simulink model "sampleModel1941_4_sub_sub_sub"  (R2023a)
settings: Solver=VariableStepAuto  StartTime=0.0  StopTime=10.0  RelTol=1e-3
libraries: hdlsllib x3, simulink x1
settings Model: Creator=user1  LastModifiedBy=user1
settings OptimizationCC: BlockReduction=off  ConditionallyExecuteInputs=off

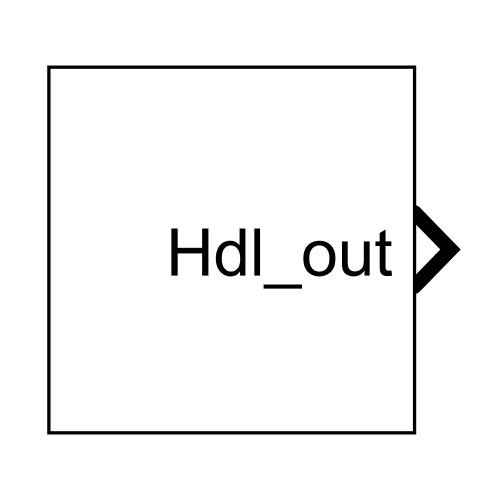
[thumbnail: Simulink's stored preview of the top-level diagram]
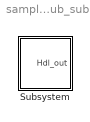
== system sampleModel1941_4_sub_sub_sub ==
  Subsystem : Subsystem

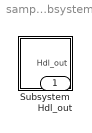
== system sampleModel1941_4_sub_sub_sub/Subsystem ==
  Subsystem : Subsystem
  Hdl_out : Outport  OutDataTypeStr=uint8

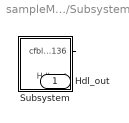
== system sampleModel1941_4_sub_sub_sub/Subsystem/Subsystem ==
  Subsystem : Subsystem
  Hdl_out : Outport  OutDataTypeStr=uint8
  wires:
  Subsystem/1(cfblk136) -> Hdl_out/1

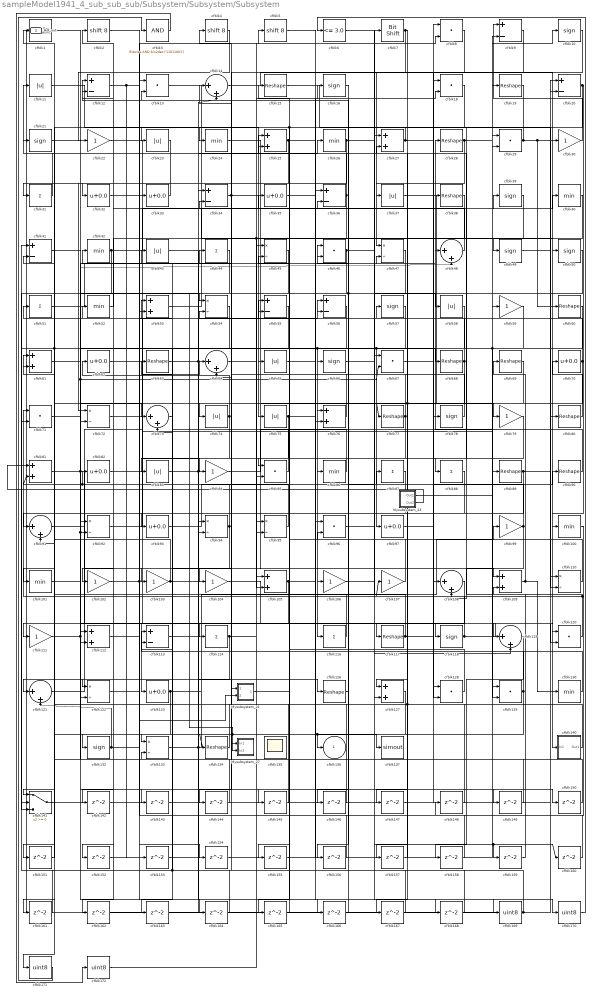
== system sampleModel1941_4_sub_sub_sub/Subsystem/Subsystem/Subsystem ==
  Mysubsystem_21 : Subsystem  TreatAsAtomicUnit=on  RTWFcnName=Mysubsystem_21
      settings: RTWFcnNameOpts=User specified  RTWFileNameOpts=Use function name
  Mysubsystem_23 : Subsystem  TreatAsAtomicUnit=on  RTWFcnName=Mysubsystem_23
      settings: RTWFcnNameOpts=User specified  RTWFileNameOpts=Use function name
  Mysubsystem_27 : Subsystem  TreatAsAtomicUnit=on  RTWFcnName=Mysubsystem_27
      settings: RTWFcnNameOpts=User specified  RTWFileNameOpts=Use function name
  cfblk1 : hdlsllib/Logic and Bit Operations/Detect Rise Nonnegative  vinit=0  OutDataTypeStr=uint8
  cfblk{10,16,21,39,49..50,57,66,78,118,132} (11 alike) : Signum
  cfblk{24,26,40,42,52,86,100..101,130} (9 alike) : MinMax  OutDataTypeStr=uint8
  cfblk{22,30,59,79,84,99,102..104,106..107,111} (12 alike) : Gain  OutDataTypeStr=uint8
  cfblk{25,27,53,61,76,81,105,109,112,127} (10 alike) : Sum  OutDataTypeStr=uint8
  cfblk{14,48,64,73,91,108,119,121} (8 alike) : Sum  Inputs=|++  OutDataTypeStr=uint8
  cfblk{11,23,37,43,58,65,74..75,83} (9 alike) : Abs  OutDataTypeStr=uint8  SaturateOnIntegerOverflow=off
  cfblk{45,47,54,72,92,94..95,110,122,133} (10 alike) : Product  Inputs=*/  OutDataTypeStr=uint8  RndMeth=Zero  SaturateOnIntegerOverflow=on
  cfblk{9,12,20,34,36,41,55..56,113} (9 alike) : Sum  Inputs=+-  OutDataTypeStr=uint8
  cfblk{31,44,51,87..88,114,116} (7 alike) : Sum  Inputs=+  OutDataTypeStr=uint8
  cfblk{15,19,28,38,60,63,68..69,77,80,89..90,117,126,134} (15 alike) : Reshape
  cfblk{8,13,18,29,46,67,71,85,96,120,128..129} (12 alike) : DotProduct  OutDataTypeStr=uint8
  cfblk{32..33,35,62,70,82,93,97,123} (9 alike) : Bias  Bias=0.0  SaturateOnIntegerOverflow=off
  cfblk135 : Scope
      settings: Floating=on
  cfblk137 : ToWorkspace  VariableName=simout  SaveFormat=Timeseries  SampleTime=-1
  cfblk140 : Subsystem
      settings: LibrarySourceBlock=|
      | hdlsllib/Ports &
      | Subsystems/Subsystem
  cfblk141 : Switch  OutDataTypeStr=uint8  SaturateOnIntegerOverflow=off  InputSameDT=off
  cfblk{142..168} (27 alike) : Delay  SampleTime=1
  cfblk{169..172} (4 alike) : DataTypeConversion  OutDataTypeStr=uint8  SaturateOnIntegerOverflow=off  RndMeth=Floor
  cfblk2 : ArithShift  BitShiftNumber=8
  cfblk3 : simulink/Logic and Bit Operations/Bitwise Operator  logicop=AND  UseBitMask=on  BitMask=bin2dec('11011001')  BitMaskRealWorld=Stored Integer
      settings: LibrarySourceBlock=|
      | hdlsllib/Logic and Bit
      | Operations/Bitwise
      | Operator
  cfblk4 : ArithShift  BitShiftNumber=8
  cfblk5 : ArithShift  BitShiftNumber=8
  cfblk6 : hdlsllib/Logic and Bit Operations/Compare To Constant  relop=<=  const=3.0  OutDataTypeStr=uint8
  cfblk7 : hdlsllib/Logic and Bit Operations/Bit Shift  mode=Shift Left Logical  N=0
  cfblk136 : Outport  OutDataTypeStr=uint8  VectorParamsAs1DForOutWhenUnconnected=off
  Hdl_out : Outport  Port=2  OutDataTypeStr=uint8
  wires:
  cfblk76/1 -> cfblk42/1
  cfblk77/1 -> cfblk85/1, cfblk12/1
  cfblk23/1 -> cfblk72/1
  cfblk118/1 -> cfblk120/1, cfblk71/1
  cfblk56/1 -> cfblk85/2, cfblk116/1
  cfblk42/1 -> cfblk19/1, cfblk71/2
  cfblk24/1 -> cfblk79/1
  cfblk32/1 -> cfblk118/1
  cfblk68/1 -> cfblk57/1, cfblk157/1, cfblk77/1
  cfblk91/1 -> cfblk103/1
  cfblk14/1 -> cfblk140/1(In1)
  cfblk70/1 -> cfblk142/1, cfblk34/2
  cfblk12/1 -> cfblk154/1, cfblk153/1
  cfblk25/1 -> cfblk119/1, cfblk111/1
  cfblk34/1 -> cfblk106/1, Mysubsystem_21/1(In1)
  cfblk116/1 -> cfblk61/1
  cfblk121/1 -> cfblk64/1
  cfblk22/1 -> cfblk84/1
  cfblk53/1 -> cfblk39/1
  cfblk4/1 -> cfblk22/1
  cfblk51/1 -> cfblk8/1
  cfblk72/1 -> cfblk128/1
  cfblk13/1 -> cfblk50/1
  cfblk45/1 -> cfblk104/1
  cfblk55/1 -> cfblk112/2
  cfblk74/1 -> cfblk83/1, cfblk62/1
  cfblk85/1 -> cfblk51/1
  cfblk52/1 -> cfblk2/1
  cfblk81/1 -> cfblk44/1, cfblk123/1
  cfblk86/1 -> cfblk52/1
  cfblk54/1 -> cfblk141/3, cfblk91/1
  cfblk130/1 -> cfblk113/1
  cfblk90/1 -> cfblk28/1
  cfblk114/1 -> cfblk8/2, cfblk121/1
  cfblk36/1 -> cfblk53/2, cfblk4/1
  cfblk134/1 -> cfblk113/2
  cfblk27/1 -> cfblk24/1, cfblk109/1
  cfblk9/1 -> cfblk47/1
  cfblk58/1 -> cfblk93/1, cfblk97/1
  cfblk11/1 -> cfblk75/1
  cfblk66/1 -> cfblk160/1, cfblk159/1
  cfblk133/1 -> cfblk166/1, cfblk38/1, cfblk99/1
  cfblk128/1 -> cfblk15/1
  cfblk126/1 -> cfblk46/1
  cfblk107/1 -> cfblk46/2
  cfblk31/1 -> cfblk11/1
  cfblk2/1 -> cfblk33/1
  cfblk83/1 -> cfblk120/2, cfblk26/1
  cfblk46/1 -> cfblk58/1, Mysubsystem_27/1(In1)
  cfblk103/1 -> cfblk41/2, cfblk25/1
  cfblk20/1 -> cfblk31/1, cfblk100/1
  cfblk26/1 -> cfblk119/2, cfblk65/1
  cfblk30/1 -> cfblk9/1
  cfblk39/1 -> cfblk132/1
  cfblk104/1 -> cfblk117/1
  cfblk123/1 -> cfblk161/1, cfblk67/1
  cfblk132/1 -> cfblk121/2, Mysubsystem_21/2(In2)
  cfblk78/1 -> cfblk13/2
  cfblk10/1 -> cfblk128/2
  cfblk48/1 -> cfblk12/2
  cfblk140/1(Out1) -> cfblk87/1, cfblk53/1
  cfblk21/1 -> cfblk66/1
  cfblk141/1 -> cfblk78/1
  cfblk106/1 -> cfblk27/1
  cfblk69/1 -> cfblk101/1
  cfblk117/1 -> cfblk90/1, cfblk55/1
  cfblk102/1 -> cfblk164/1, cfblk5/1
  cfblk84/1 -> cfblk29/1
  cfblk18/1 -> cfblk165/1, cfblk72/2
  cfblk50/1 -> cfblk171/1, cfblk76/1
  cfblk99/1 -> cfblk108/2, cfblk36/2
  cfblk59/1 -> cfblk129/2, cfblk127/1
  cfblk127/1 -> Mysubsystem_27/2(In2), cfblk134/1
  cfblk38/1 -> cfblk86/1
  cfblk79/1 -> cfblk105/2
  cfblk92/1 -> cfblk45/1
  cfblk110/1 -> cfblk35/1
  cfblk113/1 -> cfblk89/1
  cfblk37/1 -> cfblk129/1
  cfblk65/1 -> cfblk47/2
  cfblk97/1 -> cfblk108/1
  cfblk15/1 -> cfblk80/1
  cfblk80/1 -> cfblk70/1
  cfblk33/1 -> cfblk32/1
  cfblk71/1 -> cfblk114/1
  cfblk60/1 -> cfblk127/2
  cfblk129/1 -> cfblk96/2, cfblk152/1, cfblk136/1
  cfblk40/1 -> cfblk74/1, cfblk95/2
  cfblk7/1 -> cfblk64/2, cfblk37/1
  cfblk75/1 -> cfblk170/1, cfblk94/2
  cfblk105/1 -> cfblk122/2, cfblk137/1
  cfblk62/1 -> cfblk68/1
  cfblk89/1 -> cfblk141/1, cfblk30/1
  cfblk88/1 -> cfblk102/1
  cfblk61/1 -> cfblk73/1
  cfblk35/1 -> cfblk18/2
  cfblk67/1 -> cfblk40/1
  cfblk1/1 -> cfblk54/1
  cfblk6/1 -> cfblk169/1
  cfblk93/1 -> cfblk7/1
  cfblk28/1 -> cfblk167/1, cfblk10/1
  cfblk19/1 -> cfblk88/1
  cfblk29/1 -> cfblk23/1, cfblk60/1, cfblk110/2
  cfblk49/1 -> cfblk20/1
  cfblk109/1 -> cfblk130/1, cfblk69/1
  cfblk64/1 -> cfblk16/1
  cfblk73/1 -> cfblk133/1
  cfblk63/1 -> cfblk14/2, cfblk126/1
  cfblk112/1 -> cfblk56/1
  cfblk120/1 -> cfblk107/1, cfblk21/1
  cfblk111/1 -> cfblk168/1, cfblk92/2, cfblk67/2, cfblk48/2
  cfblk82/1 -> cfblk9/2
  cfblk57/1 -> cfblk122/1
  cfblk95/1 -> cfblk63/1
  cfblk96/1 -> cfblk48/1
  cfblk94/1 -> cfblk163/1, cfblk82/1, cfblk81/2
  cfblk5/1 -> cfblk49/1
  cfblk142/1 -> cfblk36/1
  cfblk101/1 -> cfblk143/1
  cfblk143/1 -> cfblk18/1
  cfblk47/1 -> cfblk144/1
  cfblk144/1 -> cfblk1/1
  cfblk122/1 -> cfblk145/1
  cfblk145/1 -> cfblk92/1
  cfblk16/1 -> cfblk146/1
  cfblk146/1 -> cfblk73/2
  cfblk8/1 -> cfblk147/1
  cfblk147/1 -> cfblk110/1
  cfblk100/1 -> cfblk148/1
  cfblk148/1 -> cfblk61/2
  cfblk41/1 -> cfblk149/1
  cfblk149/1 -> cfblk55/2
  cfblk43/1 -> cfblk150/1
  cfblk150/1 -> cfblk112/1
  cfblk108/1 -> cfblk151/1
  cfblk151/1 -> cfblk91/2
  cfblk152/1 -> cfblk95/1
  cfblk153/1 -> cfblk96/1
  cfblk154/1 -> cfblk76/2
  cfblk155/1 -> cfblk29/2
  cfblk87/1 -> cfblk156/1
  cfblk156/1 -> cfblk14/1
  cfblk157/1 -> cfblk27/2
  cfblk119/1 -> cfblk158/1
  cfblk158/1 -> cfblk13/1
  cfblk159/1 -> cfblk109/2
  cfblk160/1 -> cfblk34/1
  cfblk161/1 -> cfblk141/2
  cfblk44/1 -> cfblk162/1
  cfblk162/1 -> cfblk94/1
  cfblk163/1 -> cfblk20/2
  cfblk164/1 -> cfblk133/2
  cfblk165/1 -> cfblk45/2
  cfblk166/1 -> cfblk56/2
  cfblk167/1 -> cfblk25/2
  cfblk168/1 -> cfblk54/2
  cfblk169/1 -> Hdl_out/1, cfblk41/1, cfblk43/1
  cfblk170/1 -> cfblk6/1
  cfblk171/1 -> cfblk3/1
  cfblk3/1 -> cfblk172/1
  cfblk172/1 -> cfblk105/1
  Mysubsystem_21/1(Out1) -> cfblk155/1
  Mysubsystem_23/1(Out1) -> cfblk59/1
  Mysubsystem_23/2(Out2) -> cfblk81/1

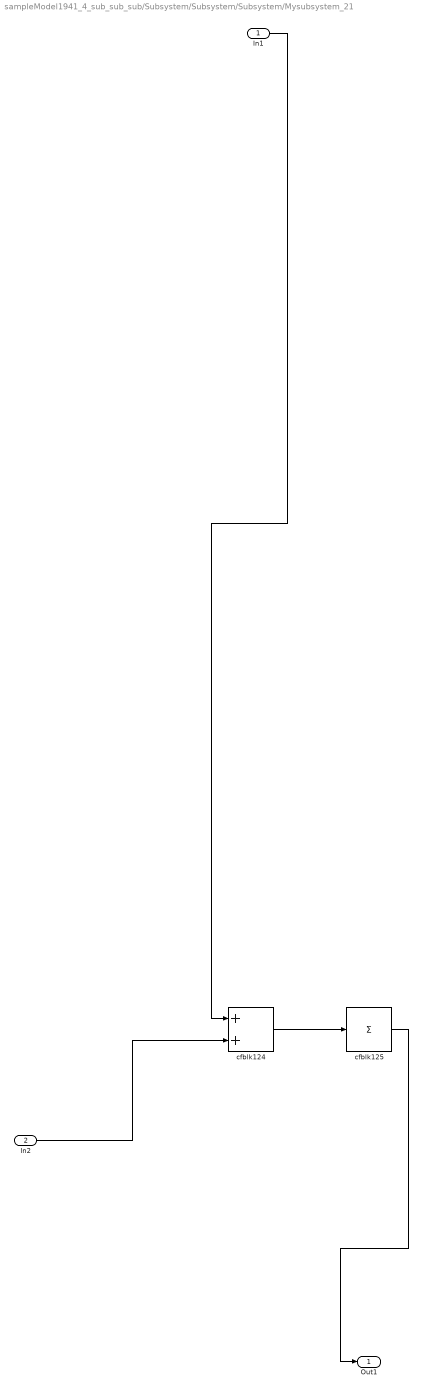
== system sampleModel1941_4_sub_sub_sub/Subsystem/Subsystem/Subsystem/Mysubsystem_21 ==
  In1 : Inport
  In2 : Inport  Port=2
  cfblk124 : Sum
  cfblk125 : Sum  Inputs=+
  Out1 : Outport
  wires:
  In1/1 -> cfblk124/1
  cfblk125/1 -> Out1/1
  In2/1 -> cfblk124/2
  cfblk124/1 -> cfblk125/1

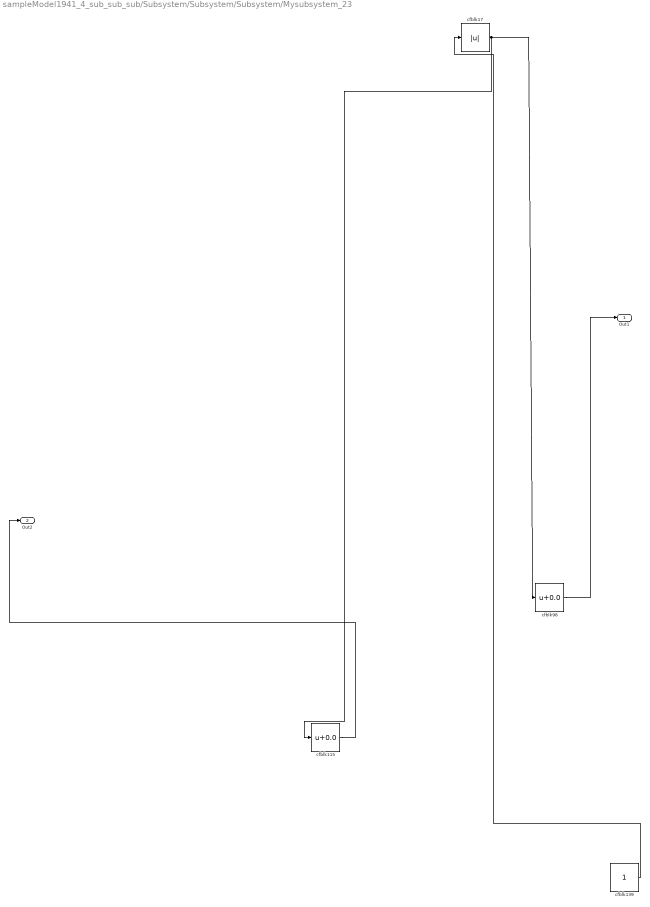
== system sampleModel1941_4_sub_sub_sub/Subsystem/Subsystem/Subsystem/Mysubsystem_23 ==
  cfblk115 : Bias  Bias=0.0  SaturateOnIntegerOverflow=off
  cfblk139 : Constant  SampleTime=-1
  cfblk17 : Abs  SaturateOnIntegerOverflow=off
  cfblk98 : Bias  Bias=0.0  SaturateOnIntegerOverflow=off
  Out1 : Outport
  Out2 : Outport  Port=2
  wires:
  cfblk98/1 -> Out1/1
  cfblk115/1 -> Out2/1
  cfblk139/1 -> cfblk17/1
  cfblk17/1 -> cfblk115/1, cfblk98/1

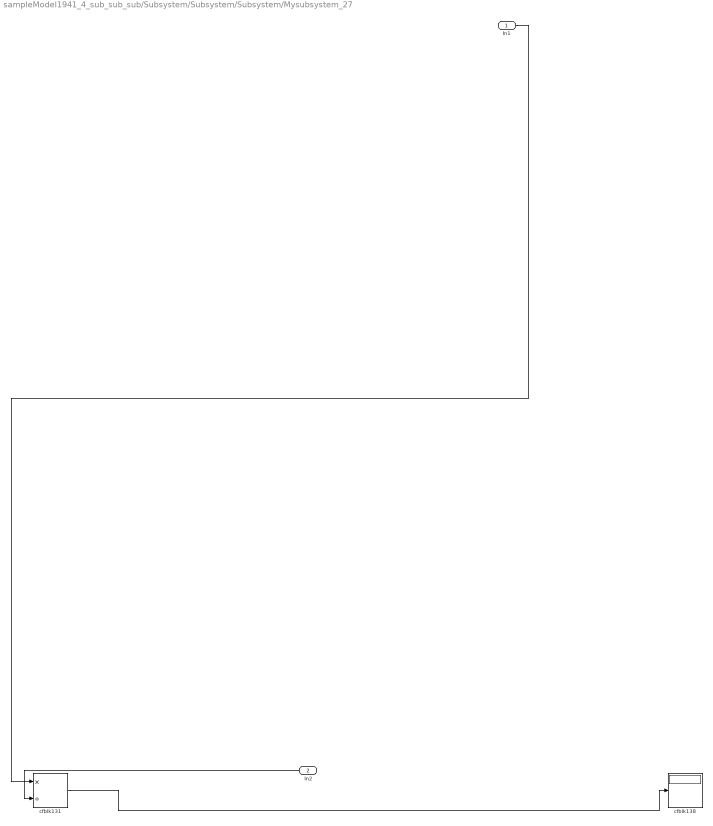
== system sampleModel1941_4_sub_sub_sub/Subsystem/Subsystem/Subsystem/Mysubsystem_27 ==
  In1 : Inport
  In2 : Inport  Port=2
  cfblk131 : Product  Inputs=*/  RndMeth=Zero  SaturateOnIntegerOverflow=on
  cfblk138 : Display
  wires:
  In1/1 -> cfblk131/1
  In2/1 -> cfblk131/2
  cfblk131/1 -> cfblk138/1

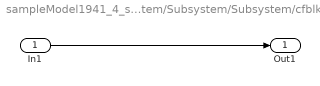
== system sampleModel1941_4_sub_sub_sub/Subsystem/Subsystem/Subsystem/cfblk140 ==
  In1 : Inport
  Out1 : Outport
  wires:
  In1/1 -> Out1/1
